simulink library "asr"  (Simulink 8.1)
settings: Solver=ode45  StartTime=0.0  StopTime=10.0  RelTol=1e-3
undefined symbols (not defined in the file or in its folder): FALSE, KJUD_AEBMaxActSpeed_kph, KJUD_AEBMaxDeactSpeed_kph, KJUD_AEBMinActSpeed_kph, KJUD_AEBMinDeactSpeed_kph, TRUE
settings Model: Creator=AT015086  LastModifiedBy=tescamilla

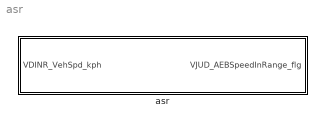
== system asr ==
  asr : Subsystem

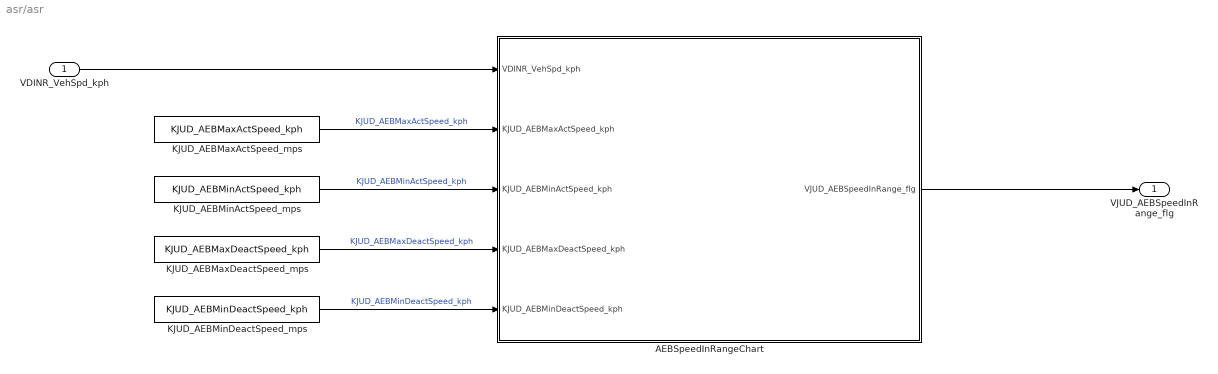
== system asr/asr ==
  "VDINR_VehSpd_kph " : Inport
  AEBSpeedInRangeChart : Stateflow chart  TreatAsAtomicUnit=on
  KJUD_AEBMaxActSpeed_mps : Constant  Value=KJUD_AEBMaxActSpeed_kph  OutDataTypeStr=single
  KJUD_AEBMaxDeactSpeed_mps : Constant  Value=KJUD_AEBMaxDeactSpeed_kph
  KJUD_AEBMinActSpeed_mps : Constant  Value=KJUD_AEBMinActSpeed_kph
  KJUD_AEBMinDeactSpeed_mps : Constant  Value=KJUD_AEBMinDeactSpeed_kph
  VJUD_AEBSpeedInRange_flg : Outport
  wires:
  "VDINR_VehSpd_kph "/1 -> AEBSpeedInRangeChart/1(VDINR_VehSpd_kph)
  AEBSpeedInRangeChart/1(VJUD_AEBSpeedInRange_flg) -> VJUD_AEBSpeedInRange_flg/1
  KJUD_AEBMinActSpeed_mps/1 -> AEBSpeedInRangeChart/3(KJUD_AEBMinActSpeed_kph)  "KJUD_AEBMinActSpeed_kph"
  KJUD_AEBMaxActSpeed_mps/1 -> AEBSpeedInRangeChart/2(KJUD_AEBMaxActSpeed_kph)  "KJUD_AEBMaxActSpeed_kph"
  KJUD_AEBMaxDeactSpeed_mps/1 -> AEBSpeedInRangeChart/4(KJUD_AEBMaxDeactSpeed_kph)  "KJUD_AEBMaxDeactSpeed_kph"
  KJUD_AEBMinDeactSpeed_mps/1 -> AEBSpeedInRangeChart/5(KJUD_AEBMinDeactSpeed_kph)  "KJUD_AEBMinDeactSpeed_kph"

== stateflow chart asr/AEBSpeedInRangeChart ==
  state SPEED_OUT_OF_RANGE
    en:
    VJUD_AEBSpeedInRange_flg=FALSE;
  state SPEED_IN_RANGE
    en:
    VJUD_AEBSpeedInRange_flg=TRUE;
  (default) -> SPEED_OUT_OF_RANGE
  SPEED_OUT_OF_RANGE -> SPEED_IN_RANGE : [(VDINR_VehSpd_kph>KJUD_AEBMinActSpeed_kph)&&...
      | (VDINR_VehSpd_kph<KJUD_AEBMaxActSpeed_kph)]
  SPEED_IN_RANGE -> SPEED_OUT_OF_RANGE : [(VDINR_VehSpd_kph<KJUD_AEBMinDeactSpeed_kph)||...
      | (VDINR_VehSpd_kph>KJUD_AEBMaxDeactSpeed_kph)]
  data: VDINR_VehSpd_kph input single; VJUD_AEBSpeedInRange_flg output boolean; FALSE parameter boolean; TRUE parameter boolean; KJUD_AEBMaxActSpeed_kph input single; KJUD_AEBMinActSpeed_kph input single; KJUD_AEBMaxDeactSpeed_kph input single; KJUD_AEBMinDeactSpeed_kph input single
